simulink model "furuta"  (R2026a)
settings: Solver=VariableStepAuto  StopTime=20.0  MaxStep=0.0001  AbsTol=1e-3  EnableMultiTasking=on
values from neighbouring files (symbols this model uses):
  g = 9.81    [main.m]
  m = 0.2    [main.m]
undefined symbols (not defined in the file or in its folder): kd_pend, ki_pend, kp_arm, kp_pend, l_arm, l_pendulum, m_arm, m_pendulum, X, Y, Z
libraries: nesl_utility x15, sm_lib x12
settings Model: Creator=pawsooon  LastModifiedBy=pawsooon
settings DebuggingCC: SubsystemReferenceDiagnosticForUnitTest=warning
settings SimscapeCC: SimscapeNominalValues="[{\"value\":\"1\",\"unit\":\"A\"},{\"value\":\"1\",\"unit\":\"bar\"},{\"value\":\"1\",\"unit\":\"cm^2\"},{\"value\":\"1\",\"unit\":\"cm^3/s\"},{\"value\":\"1\",\"unit\":\"kJ/kg\"},{\"value\":\"1\",\"unit\":\"kW\"},{\"value\":\"1\",\"unit\":\"l\"},{\"value\":\"1\",\"unit\":\"N\"},{\"value\":\"1\",\"unit\":\"N*m\"},{\"value\":\"1\",\"unit\":\"V\"}]"
settings ExplorerConfigSet: InternalSimMechanicsExplorerSettings=|
  | <ExplorerConfiguration>
  | 
  |   <canonicalview>default</canonicalview>
  | 
  |   <TilePanel>
  |     <TileInfo>
  |       <Tiles Columns="1" Count="1" Height="654" Rows="1" Width="1140">
  |         <Row Weight="1"/>
  |         <Column Weight="1"/>
  |         <Tile Height="1" Width="1" X="0" Y="0"/>
  |       </Tiles>
  |     </TileInfo>
  |     <SceneInfo>
  |       <SceneViewer>
  |         <IsThisViewStd>
  |           <IsStandardView>off</IsStandardView>
  |           <StandardViewName>Front</StandardViewName>
  |         </IsThisViewStd>
  |         <BGColor>
  |           <R>1</R>
  |           <G>1</G>
  |           <B>1</B>
  |           <A>1</A>
  |         </BGColor>
  |         <Camera>
  |           <DoPerspective>off</DoPerspective>
  |           <Position>
  |             <X>-0.66234000000000004</X>
  |             <Y>-2.58081</Y>
  |             <Z>0.40234999999999999</Z>
  |           </Position>
  |           <Center>
  |             <X>-0.27700000000000002</X>
  |             <Y>-0.072819999999999996</Y>
  |             <Z>0.019810000000000001</Z>
  |           </Center>
  |           <Up>
  |             <X>0.012930054014291247</X>
  |             <Y>0.14883024024091671</Y>
  |             <Z>0.98877822250139513</Z>
  |           </Up>
  |           <XLim>0.37220769204352794</XLim>
  |           <YLim>0.37220769204352794</YLim>
  |           <ViewLimDist>0.01</ViewLimDist>
  |         </Camera>
  |       </SceneViewer>
  |     </SceneInfo>
  |   </TilePanel>
  | 
  |   <MechEditorPanel>
  |     <GfxPanelCameraMap/>
  |     <Cameras/>
  |     <VideoCreator>
  |       <IncludeTiles>All</IncludeTiles>
  |       <IncludeTime>on</IncludeTime>
  |       <IncludeWorldFrame>off</IncludeWorldFrame>
  |       <PlaybackSpeedRatio>1</PlaybackSpeedRatio>
  |       <FrameRate>30</FrameRate>
  |       <FrameSize>auto</FrameSize>
  |       <VideoFormat>UncompressedAVI</VideoFormat>
  |     </VideoCreator>
  |   </MechEditorPanel>
  | 
  |   <PlaybackSettings>
  |     <PlaybackSpeedFactor>0.125</PlaybackSpeedFactor>
  |   </PlaybackSettings>
  | 
  | </ExplorerConfiguration>

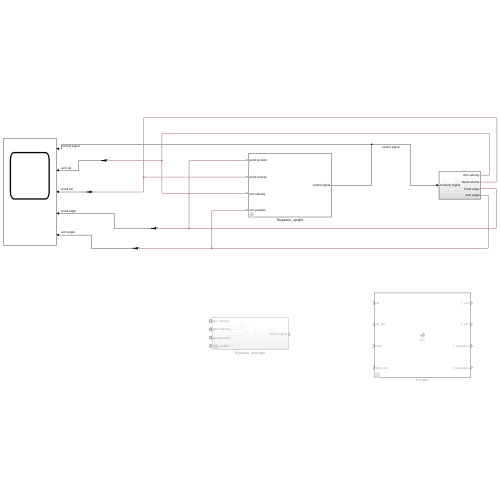
[thumbnail: Simulink's stored preview of the top-level diagram]
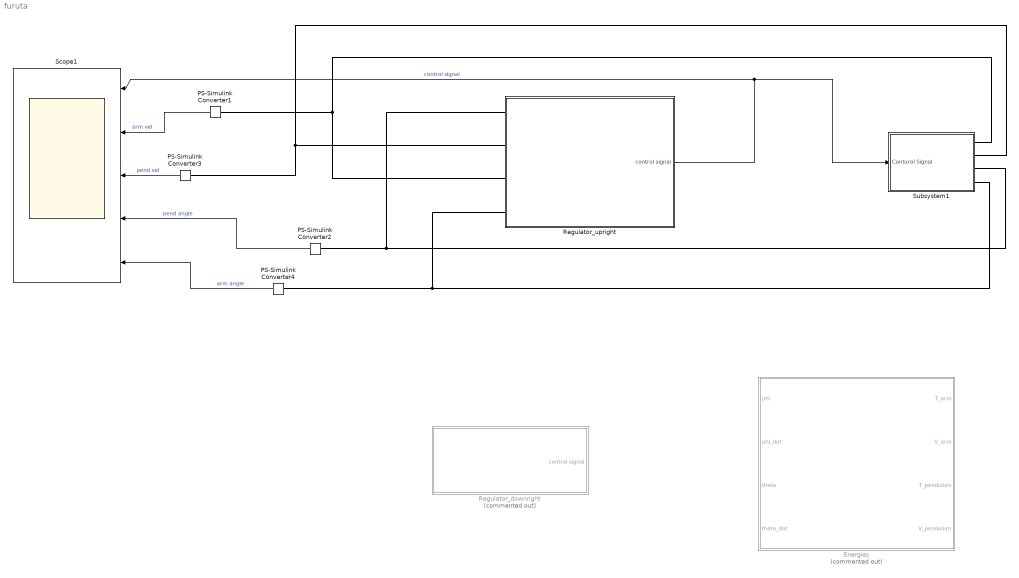
== system furuta ==
  Energies : MATLAB Function  Commented=on  TreatAsAtomicUnit=on
  PS-Simulink Converter{1..4} (4 alike) : nesl_utility/PS-Simulink Converter  PhysicalDomain=network_engine_domain  SubClassName=ps_output  LeftPortType=input  RightPortType=output  PseudoPeriodic=off  Frequencies=[]  VectorFormat=inherit  Unit=inherit  AffineConversion=off
  Regulator_downright : Subsystem  Commented=on
  Regulator_upright : Subsystem  mask{kd_pend=1.4, kp_pend=25, kd_arm=0.02, kp_arm=0.06}
  Scope1 : Scope  NumInputPorts=5
      settings: ActiveDisplayYMinimum=-25  ActiveDisplayYMaximum=25  DataLoggingVariableName=ScopeData4
  Subsystem1 : Subsystem
  wires:
  Regulator_upright/1(control signal) -> Subsystem1/1(Contorol Signal), Scope1/1  "control signal"
  PS-Simulink Converter1/1 -> Scope1/2  "arm vel"
  PS-Simulink Converter3/1 -> Scope1/3  "pend vel"
  PS-Simulink Converter2/1 -> Scope1/4  "pend angle"
  PS-Simulink Converter4/1 -> Scope1/5  "arm angle"
  connections:
  Subsystem1/RConn4 -- Regulator_upright/LConn4 -- PS-Simulink Converter4/LConn1
  PS-Simulink Converter3/LConn1 -- Subsystem1/RConn2 -- Regulator_upright/LConn2
  Subsystem1/RConn1 -- Regulator_upright/LConn3 -- PS-Simulink Converter1/LConn1
  Subsystem1/RConn3 -- PS-Simulink Converter2/LConn1 -- Regulator_upright/LConn1

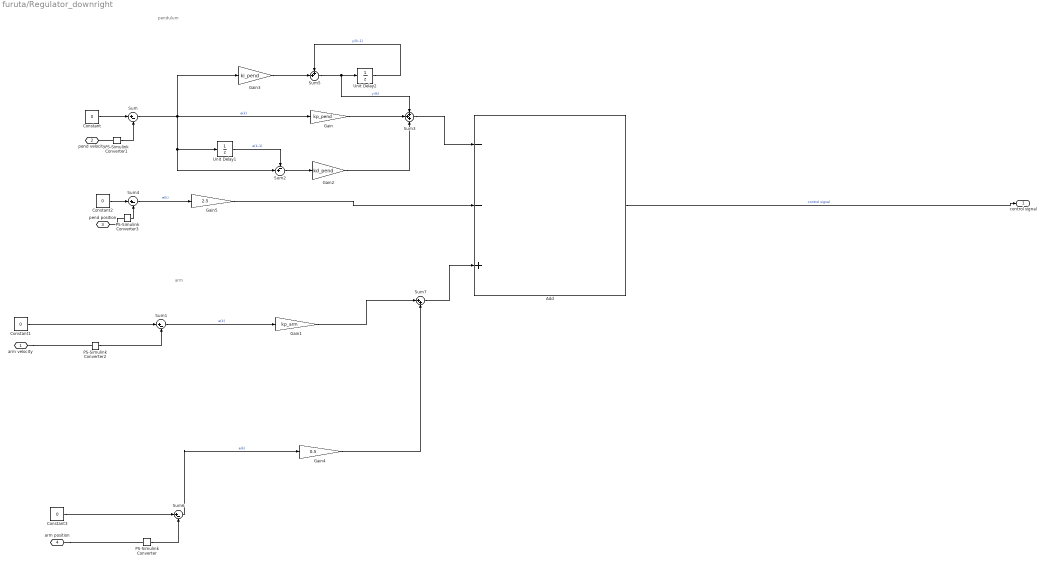
== system furuta/Regulator_downright ==
  note: pendulum
  note: arm
  Add : Sum  Inputs=--+
  Constant{,1..3} (4 alike) : Constant  Value=0
  Gain : Gain  Gain=kp_pend
  Gain1 : Gain  Gain=kp_arm
  Gain2 : Gain  Gain=kd_pend
  Gain3 : Gain  Gain=ki_pend
  Gain4 : Gain  Gain=0.5
  Gain5 : Gain  Gain=2.5
  PS-Simulink Converter{,1..3} (4 alike) : nesl_utility/PS-Simulink Converter  PhysicalDomain=network_engine_domain  SubClassName=ps_output  LeftPortType=input  RightPortType=output  PseudoPeriodic=off  Frequencies=[]  VectorFormat=inherit  Unit=inherit  AffineConversion=off
  Sum{,1,4,6} (4 alike) : Sum  Inputs=|+-
  Sum2 : Sum  Inputs=-+|
  Sum3 : Sum  Inputs=+++
  Sum5 : Sum  Inputs=++|
  Sum7 : Sum  Inputs=|++
  Unit Delay1 : UnitDelay  SampleTime=0.01
  Unit Delay2 : UnitDelay  SampleTime=0.01
  "arm velocity " : PMIOPort  Side=Left
  pend velocity : PMIOPort  Port=2  Side=Left
  pend position : PMIOPort  Port=3  Side=Left
  arm position : PMIOPort  Port=4  Side=Left
  control signal : Outport
  wires:
  Add/1 -> control signal/1  "control signal"
  Gain1/1 -> Sum7/1
  PS-Simulink Converter1/1 -> Sum/2
  Constant1/1 -> Sum1/1
  Constant/1 -> Sum/1
  PS-Simulink Converter2/1 -> Sum1/2
  Sum1/1 -> Gain1/1  "e(k)"
  Sum2/1 -> Gain2/1
  Unit Delay1/1 -> Sum2/1  "e(k-1)"
  Sum/1 -> Gain3/1, Sum2/2, Unit Delay1/1, Gain/1  "e(k)"
  Gain/1 -> Sum3/2
  Sum3/1 -> Add/1
  Gain2/1 -> Sum3/3
  Constant2/1 -> Sum4/1
  PS-Simulink Converter3/1 -> Sum4/2
  Unit Delay2/1 -> Sum5/1  "yi(k-1)"
  Gain3/1 -> Sum5/2
  Sum5/1 -> Sum3/1, Unit Delay2/1  "yi(k)"
  Constant3/1 -> Sum6/1
  Sum6/1 -> Gain4/1  "e(k)"
  PS-Simulink Converter/1 -> Sum6/2
  Sum7/1 -> Add/3
  Gain4/1 -> Sum7/2
  Sum4/1 -> Gain5/1  "e(k)"
  Gain5/1 -> Add/2
  connections:
  PS-Simulink Converter1/LConn1 -- pend velocity/RConn1
  "arm velocity "/RConn1 -- PS-Simulink Converter2/LConn1
  PS-Simulink Converter3/LConn1 -- pend position/RConn1
  arm position/RConn1 -- PS-Simulink Converter/LConn1

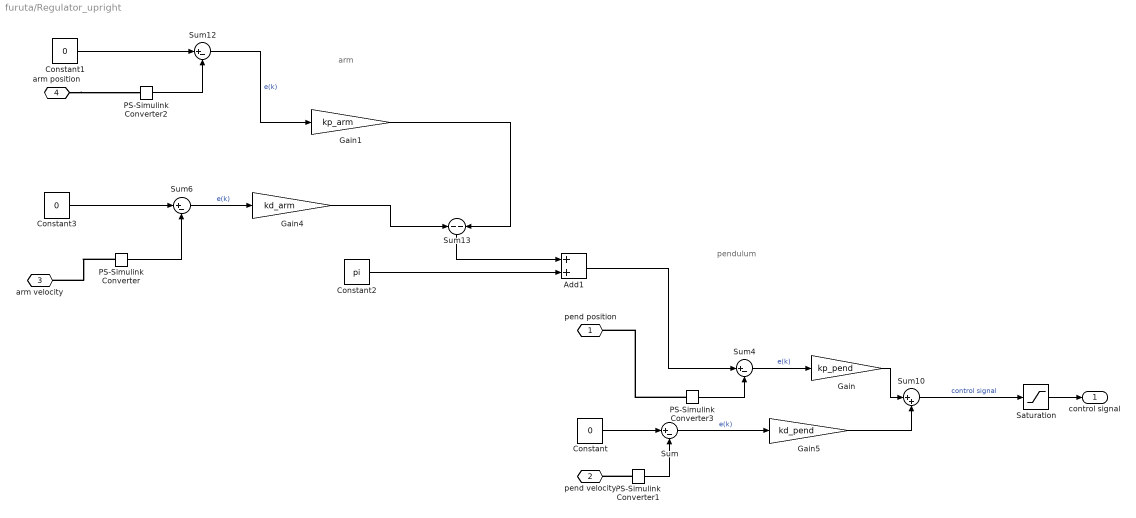
== system furuta/Regulator_upright ==
  note: pendulum
  note: arm
  Add1 : Sum
  Constant : Constant  Value=0
  Constant1 : Constant  Value=0
  Constant2 : Constant  Value=pi
  Constant3 : Constant  Value=0
  Gain : Gain  Gain=kp_pend
  Gain1 : Gain  Gain=kp_arm
  Gain4 : Gain  Gain=kd_arm
  Gain5 : Gain  Gain=kd_pend
  PS-Simulink Converter{,1..3} (4 alike) : nesl_utility/PS-Simulink Converter  PhysicalDomain=network_engine_domain  SubClassName=ps_output  LeftPortType=input  RightPortType=output  PseudoPeriodic=off  Frequencies=[]  VectorFormat=inherit  Unit=inherit  AffineConversion=off
  Saturation : Saturate  UpperLimit=20  LowerLimit=-20
  Sum{,4,6,12} (4 alike) : Sum  Inputs=|+-
  Sum10 : Sum  Inputs=|++
  Sum13 : Sum  Inputs=-|-
  pend position : PMIOPort  Side=Left
  pend velocity : PMIOPort  Port=2  Side=Left
  "arm velocity " : PMIOPort  Port=3  Side=Left
  arm position : PMIOPort  Port=4  Side=Left
  control signal : Outport
  wires:
  Sum10/1 -> Saturation/1  "control signal"
  Constant2/1 -> Add1/2
  PS-Simulink Converter3/1 -> Sum4/2
  Sum4/1 -> Gain/1  "e(k)"
  Constant/1 -> Sum/1
  PS-Simulink Converter1/1 -> Sum/2
  Sum/1 -> Gain5/1  "e(k)"
  Gain5/1 -> Sum10/2
  Add1/1 -> Sum4/1
  Sum6/1 -> Gain4/1  "e(k)"
  PS-Simulink Converter/1 -> Sum6/2
  Constant3/1 -> Sum6/1
  Constant1/1 -> Sum12/1
  PS-Simulink Converter2/1 -> Sum12/2
  Sum12/1 -> Gain1/1  "e(k)"
  Gain1/1 -> Sum13/2
  Gain4/1 -> Sum13/1
  Sum13/1 -> Add1/1
  Gain/1 -> Sum10/1
  Saturation/1 -> control signal/1
  connections:
  PS-Simulink Converter3/LConn1 -- pend position/RConn1
  PS-Simulink Converter1/LConn1 -- pend velocity/RConn1
  PS-Simulink Converter/LConn1 -- "arm velocity "/RConn1
  arm position/RConn1 -- PS-Simulink Converter2/LConn1

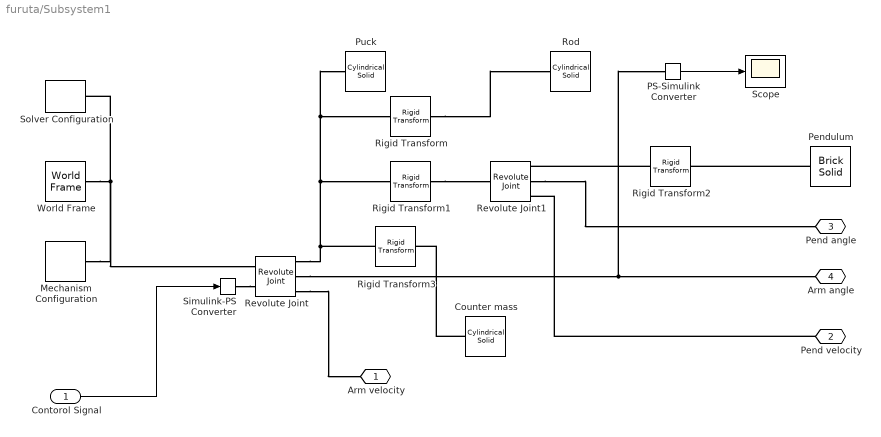
== system furuta/Subsystem1 ==
  Contorol Signal : Inport
  Counter mass : sm_lib/Body Elements/Cylindrical Solid  CylinderRadius=0.075/2  CylinderRadiusUnits=m  CylinderLength=0.025  CylinderLengthUnits=m  ExportEntireGeometry=off  InertiaType=CalculateFromGeometry  BasedOnType=Mass  Density=2.7  DensityUnits=g/cm^3  Mass=0.4  MassUnits=kg  CenterOfMass=[0 0 0]  CenterOfMassUnits=m  MomentsOfInertia=[1 1 1]  MomentsOfInertiaUnits=kg*m^2  ProductsOfInertia=[0 0 0]  ProductsOfInertiaUnits=kg*m^2  GraphicType=FromGeometry  MarkerShape=Sphere  MarkerSize=10  GraphicVisPropType=AdvancedVisualProperties  GraphicDiffuseColor=[1 0 0]  GraphicOpacity=1  GraphicSpecularColor=[0.5 0.5 0.5 1.0]  GraphicAmbientColor=[0.15 0.15 0.15 1.0]  GraphicEmissiveColor=[0.0 0.0 0.0 1.0]  GraphicShininess=75  DoExposeReferenceFrame=on  SerializedFrames=<Frames/>
  Mechanism Configuration : sm_lib/Utilities/Mechanism Configuration  UniformGravity=Constant  GravityVector=[0 0 -9.80665]  GravityVectorUnits=m/s^2  LinearizationDelta=0.001  JointModeTransitionNonlinearIterations=2
  PS-Simulink Converter : nesl_utility/PS-Simulink Converter  PhysicalDomain=network_engine_domain  SubClassName=ps_output  LeftPortType=input  RightPortType=output  PseudoPeriodic=off  Frequencies=[]  VectorFormat=inherit  Unit=inherit  AffineConversion=off
  Pendulum : sm_lib/Body Elements/Brick Solid  BrickDimensions=[2.5 1.0 60]  BrickDimensionsUnits=cm  ExportEntireGeometry=off  InertiaType=CalculateFromGeometry  BasedOnType=Density  Density=2.7  DensityUnits=g/cm^3  Mass=1  MassUnits=kg  CenterOfMass=[0 0 0]  CenterOfMassUnits=m  MomentsOfInertia=[1 1 1]  MomentsOfInertiaUnits=kg*m^2  ProductsOfInertia=[0 0 0]  ProductsOfInertiaUnits=kg*m^2  GraphicType=FromGeometry  MarkerShape=Sphere  MarkerSize=10  GraphicVisPropType=SimpleVisualProperties  GraphicDiffuseColor=[0.5 0.5 0.5]  GraphicOpacity=1  GraphicSpecularColor=[0.5 0.5 0.5 1.0]  GraphicAmbientColor=[0.15 0.15 0.15 1.0]  GraphicEmissiveColor=[0.0 0.0 0.0 1.0]  GraphicShininess=75  DoExposeReferenceFrame=on  SerializedFrames=<Frames/>
  Puck : sm_lib/Body Elements/Cylindrical Solid  CylinderRadius=0.075/2  CylinderRadiusUnits=m  CylinderLength=0.025  CylinderLengthUnits=m  ExportEntireGeometry=off  InertiaType=CalculateFromGeometry  BasedOnType=Density  Density=2.7  DensityUnits=g/cm^3  Mass=1  MassUnits=kg  CenterOfMass=[0 0 0]  CenterOfMassUnits=m  MomentsOfInertia=[1 1 1]  MomentsOfInertiaUnits=kg*m^2  ProductsOfInertia=[0 0 0]  ProductsOfInertiaUnits=kg*m^2  GraphicType=FromGeometry  MarkerShape=Sphere  MarkerSize=10  GraphicVisPropType=AdvancedVisualProperties  GraphicDiffuseColor=[0 0.6667 0]  GraphicOpacity=1  GraphicSpecularColor=[0.5 0.5 0.5 1.0]  GraphicAmbientColor=[0.15 0.15 0.15 1.0]  GraphicEmissiveColor=[0.0 0.0 0.0 1.0]  GraphicShininess=75  DoExposeReferenceFrame=on  SerializedFrames=<Frames/>
  Revolute Joint : sm_lib/Joints/Revolute Joint  JointMode=Normal  CompositeWrenchDir=FollowerOnBase  CompositeWrenchFrame=BaseFrame  SenseConstraintForce=off  SenseConstraintTorque=off  SenseTotalForce=off  SenseTotalTorque=off  PositionTargetSpecify=off  PositionTargetPriority=High  PositionTargetValue=0  PositionTargetValueUnits=deg  VelocityTargetSpecify=off  VelocityTargetPriority=High  VelocityTargetValue=0  VelocityTargetValueUnits=deg/s  EquilibriumPosition=0  EquilibriumPositionUnits=deg  SpringStiffness=0  SpringStiffnessUnits=N*m/deg  DampingCoefficient=0.0005  DampingCoefficientUnits=N*m/(deg/s)  LowerLimitSpecify=off  LowerLimitBound=-90  LowerLimitBoundUnits=deg  LowerLimitStiffness=1e4  LowerLimitStiffnessUnits=N*m/deg  LowerLimitDamping=10  LowerLimitDampingUnits=N*m/(deg/s)  LowerLimitTransitionRegionWidth=0.1  LowerLimitTransitionRegionWidthUnits=deg  UpperLimitSpecify=off  UpperLimitBound=90  UpperLimitBoundUnits=deg  UpperLimitStiffness=1e4  UpperLimitStiffnessUnits=N*m/deg  UpperLimitDamping=10  UpperLimitDampingUnits=N*m/(deg/s)  UpperLimitTransitionRegionWidth=0.1  UpperLimitTransitionRegionWidthUnits=deg  TorqueActuationMode=InputTorque  MotionActuationMode=ComputedMotion  SensePosition=on  SenseVelocity=on  SenseAcceleration=off  SenseTorqueForce=off  SenseLowerLimitTorqueForce=off  SenseUpperLimitTorqueForce=off
  Revolute Joint1 : sm_lib/Joints/Revolute Joint  JointMode=Normal  CompositeWrenchDir=FollowerOnBase  CompositeWrenchFrame=BaseFrame  SenseConstraintForce=off  SenseConstraintTorque=off  SenseTotalForce=off  SenseTotalTorque=off  PositionTargetSpecify=on  PositionTargetPriority=High  PositionTargetValue=pi+0.5  PositionTargetValueUnits=rad  VelocityTargetSpecify=off  VelocityTargetPriority=High  VelocityTargetValue=0  VelocityTargetValueUnits=deg/s  EquilibriumPosition=0  EquilibriumPositionUnits=deg  SpringStiffness=0  SpringStiffnessUnits=N*m/deg  DampingCoefficient=0.0005  DampingCoefficientUnits=N*m/(deg/s)  LowerLimitSpecify=off  LowerLimitBound=-90  LowerLimitBoundUnits=deg  LowerLimitStiffness=1e4  LowerLimitStiffnessUnits=N*m/deg  LowerLimitDamping=10  LowerLimitDampingUnits=N*m/(deg/s)  LowerLimitTransitionRegionWidth=0.1  LowerLimitTransitionRegionWidthUnits=deg  UpperLimitSpecify=off  UpperLimitBound=90  UpperLimitBoundUnits=deg  UpperLimitStiffness=1e4  UpperLimitStiffnessUnits=N*m/deg  UpperLimitDamping=10  UpperLimitDampingUnits=N*m/(deg/s)  UpperLimitTransitionRegionWidth=0.1  UpperLimitTransitionRegionWidthUnits=deg  TorqueActuationMode=NoTorque  MotionActuationMode=ComputedMotion  SensePosition=on  SenseVelocity=on  SenseAcceleration=off  SenseTorqueForce=off  SenseLowerLimitTorqueForce=off  SenseUpperLimitTorqueForce=off
  Rigid Transform : sm_lib/Frames and Transforms/Rigid Transform  RotationMethod=StandardAxis  FollAlignAxisA=+X  BaseAlignAxisA=+Y  FollAlignAxisB=+Y  BaseAlignAxisB=+Z  RotationStandardAxis=+X  RotationAngle=90  RotationAngleUnits=deg  RotationArbitraryAxis=[0 0 1]  RotationSequenceAxes=FollowerAxes  RotationSequence=XYX  RotationSequenceAngles=[0 0 0]  RotationSequenceAnglesUnits=deg  RotationMatrix=[1 0 0;0 1 0;0 0 1]  Quaternion=[1 0 0 0]  TranslationMethod=None  TranslationCartesianOffset=[0 0 0]  TranslationCartesianOffsetUnits=m  TranslationStandardAxis=+Z  TranslationStandardOffset=0  TranslationStandardOffsetUnits=m  TranslationROffset=0  TranslationROffsetUnits=m  TranslationThetaOffset=0  TranslationThetaOffsetUnits=deg  TranslationZOffset=0  TranslationZOffsetUnits=m
  Rigid Transform1 : sm_lib/Frames and Transforms/Rigid Transform  RotationMethod=StandardAxis  FollAlignAxisA=+X  BaseAlignAxisA=+Y  FollAlignAxisB=+Y  BaseAlignAxisB=+Z  RotationStandardAxis=-X  RotationAngle=90  RotationAngleUnits=deg  RotationArbitraryAxis=[0 0 1]  RotationSequenceAxes=BaseAxes  RotationSequence=XYX  RotationSequenceAngles=[0 0 0]  RotationSequenceAnglesUnits=deg  RotationMatrix=[1 0 0;0 1 0;0 0 1]  Quaternion=[1 0 0 0]  TranslationMethod=StandardAxis  TranslationCartesianOffset=[0 0 0]  TranslationCartesianOffsetUnits=m  TranslationStandardAxis=+Y  TranslationStandardOffset=0.3  TranslationStandardOffsetUnits=m  TranslationROffset=0.3  TranslationROffsetUnits=m  TranslationThetaOffset=90  TranslationThetaOffsetUnits=deg  TranslationZOffset=0  TranslationZOffsetUnits=m
  Rigid Transform2 : sm_lib/Frames and Transforms/Rigid Transform  RotationMethod=StandardAxis  FollAlignAxisA=+X  BaseAlignAxisA=+Y  FollAlignAxisB=+Y  BaseAlignAxisB=+Z  RotationStandardAxis=+X  RotationAngle=90  RotationAngleUnits=deg  RotationArbitraryAxis=[0 0 1]  RotationSequenceAxes=FollowerAxes  RotationSequence=XYX  RotationSequenceAngles=[0 0 0]  RotationSequenceAnglesUnits=deg  RotationMatrix=[1 0 0;0 1 0;0 0 1]  Quaternion=[1 0 0 0]  TranslationMethod=StandardAxis  TranslationCartesianOffset=[0 0 0]  TranslationCartesianOffsetUnits=m  TranslationStandardAxis=+Y  TranslationStandardOffset=0.6/2  TranslationStandardOffsetUnits=m  TranslationROffset=0  TranslationROffsetUnits=m  TranslationThetaOffset=0  TranslationThetaOffsetUnits=deg  TranslationZOffset=0  TranslationZOffsetUnits=m
  Rigid Transform3 : sm_lib/Frames and Transforms/Rigid Transform  RotationMethod=StandardAxis  FollAlignAxisA=+X  BaseAlignAxisA=+Y  FollAlignAxisB=+Y  BaseAlignAxisB=+Z  RotationStandardAxis=+X  RotationAngle=90  RotationAngleUnits=deg  RotationArbitraryAxis=[0 0 1]  RotationSequenceAxes=BaseAxes  RotationSequence=XYX  RotationSequenceAngles=[0 0 0]  RotationSequenceAnglesUnits=deg  RotationMatrix=[1 0 0;0 1 0;0 0 1]  Quaternion=[1 0 0 0]  TranslationMethod=StandardAxis  TranslationCartesianOffset=[0 0 0]  TranslationCartesianOffsetUnits=m  TranslationStandardAxis=-Y  TranslationStandardOffset=0.3  TranslationStandardOffsetUnits=m  TranslationROffset=0.3  TranslationROffsetUnits=m  TranslationThetaOffset=90  TranslationThetaOffsetUnits=deg  TranslationZOffset=0  TranslationZOffsetUnits=m
  Rod : sm_lib/Body Elements/Cylindrical Solid  CylinderRadius=0.015/2  CylinderRadiusUnits=m  CylinderLength=0.6  CylinderLengthUnits=m  ExportEntireGeometry=off  InertiaType=CalculateFromGeometry  BasedOnType=Density  Density=2.7  DensityUnits=g/cm^3  Mass=1  MassUnits=kg  CenterOfMass=[0 0 0]  CenterOfMassUnits=m  MomentsOfInertia=[1 1 1]  MomentsOfInertiaUnits=kg*m^2  ProductsOfInertia=[0 0 0]  ProductsOfInertiaUnits=kg*m^2  GraphicType=FromGeometry  MarkerShape=Sphere  MarkerSize=10  GraphicVisPropType=SimpleVisualProperties  GraphicDiffuseColor=[0 0.6667 0]  GraphicOpacity=1  GraphicSpecularColor=[0.5 0.5 0.5 1.0]  GraphicAmbientColor=[0.15 0.15 0.15 1.0]  GraphicEmissiveColor=[0.0 0.0 0.0 1.0]  GraphicShininess=75  DoExposeReferenceFrame=on  SerializedFrames=<Frames/>
  Scope : Scope
      settings: ActiveDisplayYMinimum=-3.752857627636605  ActiveDisplayYMaximum=0.41698418084851158
  Simulink-PS Converter : nesl_utility/Simulink-PS Converter  PhysicalDomain=network_engine_domain  SubClassName=ps_input  LeftPortType=input  RightPortType=output  PseudoPeriodic=off  Frequencies=[]  NoiseDistribution=none  NoiseParameters=[]  Unit=1  AffineConversion=off  FilteringAndDerivatives=provide  SimscapeFilterOrder=1  InputFilterTimeConstant=0.001  UdotUserProvided=0
  Solver Configuration : nesl_utility/Solver Configuration  PhysicalDomain=network_engine_domain  SubClassName=solver  LeftPortType=input  RightPortType=generic  Tones=[]  Harmonics=[]  SimulateNoise=off  Profile=off  UseLocalSampling=off  EnableSwitchedLinearOptims=on  FrequencyDomain=off  UseCCode=off  RelTol=0.001  AbsTol=1e-06  MinStep=1e-09  ToWorkspace=off  RevertToSquareIcSolve=off  NumHomotopyIterations=100  PhasorMode=off  PhasorModeNumHarmonics=1  ConsistencySolver=NEWTON_XTOL_AFTER_FTOL  CanonicalOrdering=UNORDERED  OptimizeIntermediates=UNOPTIMIZED  IndexReductionMethod=DerivativeReplacement  DoDC=off  ResidualTolerance=1e-09  ConsistencyTolSource=GLOBAL  ConsistencyAbsTol=0.001  ConsistencyRelTol=0.001  ConsistencyTolFactor=0.001  UseLocalSolver=off  LocalSolverChoice=NE_BACKWARD_EULER_ADVANCER  ResolveIndetEquations=on  FunctionEvalNumThread=1  LocalSolverSampleTime=0.001  DoFixedCost=off  MaxNonlinIter=3  MaxModeIter=2  ComputeImpulses=off  ImpulseIterations=2  LinearAlgebra=Sparse  LinearAlgebraNumThread=0  EquationFormulation=NE_TIME_EF  DelaysMemoryBudget=1024  AutomaticFiltering=on  FilteringTimeConstant=0.001  PartitionStorageMethod=AS_NEEDED  PartitionMemoryBudget=1024  PartitionMethod=FAST  MultibodyUseLocalSolver=off  MultibodyLocalSolverChoice=ODE1  MultibodyLocalSolverSampleTime=0.001
  World Frame : sm_lib/Frames and Transforms/World Frame
  Arm velocity : PMIOPort  Side=Right
  Pend velocity : PMIOPort  Port=2  Side=Right
  Pend angle : PMIOPort  Port=3  Side=Right
  Arm angle : PMIOPort  Port=4  Side=Right
  wires:
  PS-Simulink Converter/1 -> Scope/1
  Contorol Signal/1 -> Simulink-PS Converter/1
  connections:
  Revolute Joint/RConn3 -- Arm velocity/RConn1
  Rigid Transform/RConn1 -- Rod/RConn1
  Rigid Transform2/LConn1 -- Revolute Joint1/RConn1
  Pend velocity/RConn1 -- Revolute Joint1/RConn3
  World Frame/RConn1 -- Mechanism Configuration/RConn1 -- Revolute Joint/LConn1 -- Solver Configuration/RConn1
  Pendulum/RConn1 -- Rigid Transform2/RConn1
  Revolute Joint/RConn2 -- Arm angle/RConn1 -- PS-Simulink Converter/LConn1
  Counter mass/RConn1 -- Rigid Transform3/RConn1
  Revolute Joint/RConn1 -- Rigid Transform3/LConn1 -- Rigid Transform1/LConn1 -- Puck/RConn1 -- Rigid Transform/LConn1
  Revolute Joint1/RConn2 -- Pend angle/RConn1
  Rigid Transform1/RConn1 -- Revolute Joint1/LConn1
  Simulink-PS Converter/RConn1 -- Revolute Joint/LConn2

== matlab function furuta/Energies ==
  data: phi input; phi_dot input; theta input; theta_dot input; T_arm output; V_arm output; T_pendulum output; V_pendulum output; g parameter; m_arm parameter; l_arm parameter; m_pendulum parameter; l_pendulum parameter
function [T_arm, V_arm, T_pendulum, V_pendulum] = fcn(phi, phi_dot, theta, theta_dot, g, m_arm, l_arm, m_pendulum, l_pendulum)

% dane m, l, g itp. trzeba zczytac z wlasciwosci modelu w srodku

% Horizontal arm
T_arm = 0.5 * 1/3 * m_arm * l_arm^2 * phi_dot;
V_arm = 0;


% Pendulum arm
T_pendulum = 0.5 * m_pendulum * (l_arm^2 + 1/3 * l_pendulum^2 * sin(theta)^2) * phi_dot^2 + m_pendulum * l_arm * l_pendulum * cos(theta) * phi_dot * theta_dot + 1/3 * m_pendulum * l_pendulum^2 * theta_dot^2;
V_pendulum = 0.5 * m_pendulum * g * l_pendulum * cos(theta);
